simulink model "modelo_sim"  (R2022b)
settings: Solver=VariableStepAuto  StartTime=0.0  StopTime=20  RelTol=1e-3
values from neighbouring files (symbols this model uses):
  b1 = 10    [modelo.m]
  b2 = 10    [modelo.m]
  f = 2000    [modelo.m]
  k = 10    [modelo.m]
  m1 = 400    [modelo.m]
  m2 = 10000    [modelo.m]
settings Model: Creator=Fran  LastModifiedBy=Fran

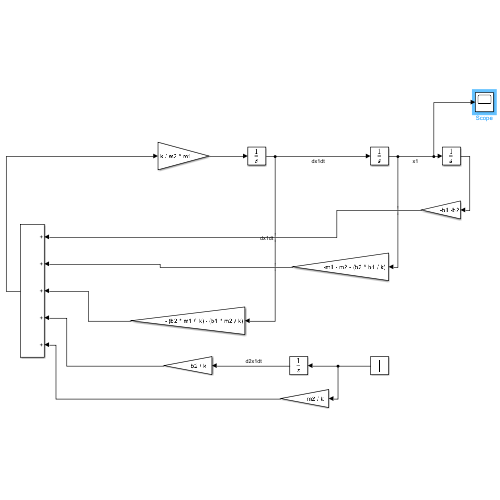
[thumbnail: Simulink's stored preview of the top-level diagram]
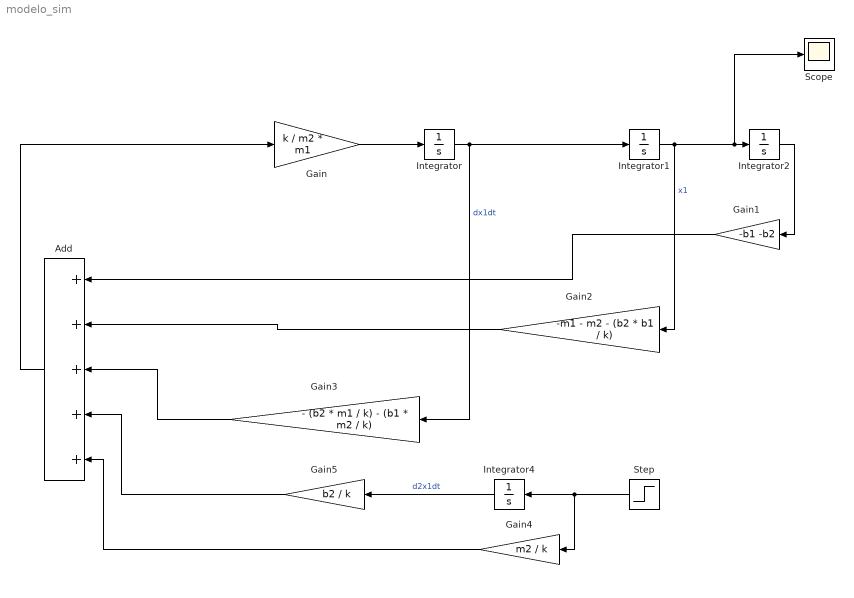
== system modelo_sim ==
  Add : Sum  Inputs=+++++
  Gain : Gain  Gain=k / m2 * m1
  Gain1 : Gain  Gain=-b1 -b2
  Gain2 : Gain  Gain=-m1 - m2 - (b2 * b1 / k)
  Gain3 : Gain  Gain="- (b2 * m1 /  k) - (b1 * m2 / k)"
  Gain4 : Gain  Gain=m2 / k
  Gain5 : Gain  Gain=b2 / k
  Integrator{,1..2,4} (4 alike) : Integrator
  Scope : Scope
  Step : Step  After=f  SampleTime=0
  wires:
  Integrator2/1 -> Gain1/1
  Integrator1/1 -> Gain2/1, Scope/1, Integrator2/1  "x1"
  Integrator/1 -> Gain3/1, Integrator1/1  "dx1dt"
  Gain/1 -> Integrator/1
  Step/1 -> Gain4/1, Integrator4/1
  Integrator4/1 -> Gain5/1  "d2x1dt"
  Gain1/1 -> Add/1
  Gain2/1 -> Add/2
  Gain3/1 -> Add/3
  Gain5/1 -> Add/4
  Gain4/1 -> Add/5
  Add/1 -> Gain/1
